simulink model "washout2useful"  (R2018b)
settings: Solver=VariableStepAuto  StartTime=0.0  StopTime=30  RelTol=1e-3
undefined symbols (not defined in the file or in its folder): sigbuilder_block
settings Model: Creator=15705  LastModifiedBy=15705

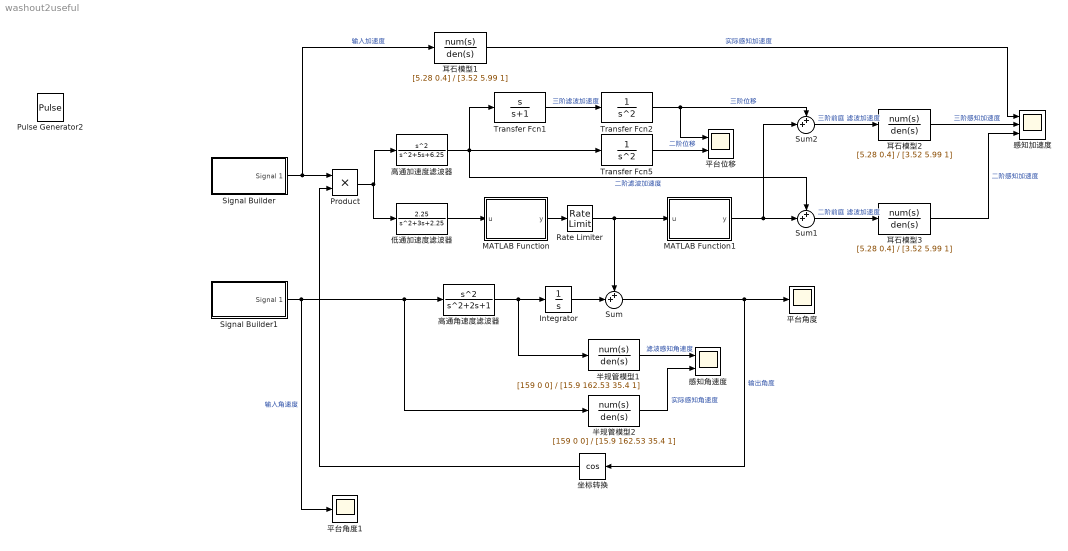
== system washout2useful ==
  Integrator : Integrator
  MATLAB Function : MATLAB Function  TreatAsAtomicUnit=on
  MATLAB Function1 : MATLAB Function  TreatAsAtomicUnit=on
  Product : Product
  Pulse Generator2 : DiscretePulseGenerator  PulseType=Time based  Period=10  PulseWidth=50  PhaseDelay=2
  Rate Limiter : RateLimiter  RisingSlewLimit=0.0628  FallingSlewLimit=-0.0628  SampleTimeMode=inherited
  Signal Builder : Subsystem  Tag=STV Subsys  LoadFcn=sigbuilder_block('load');  StartFcn=sigbuilder_block('start');  StopFcn=sigbuilder_block('stop');  ClipboardFcn=sigbuilder_block('clipboard');  mask(Sigbuilder block){tuvar=[0:10]}
      mask help: Simulink:masks:SigbuilderBlock_MD
      mask init:
      | if ~strcmp(get_param(bdroot(gcbh),'SimulationStatus'),'stopped') tuvar = sigbuilder_block('maskInit'); end
      settings: CopyFcn=sigbuilder_block('copy');  DeleteFcn=sigbuilder_block('delete');  ModelCloseFcn=sigbuilder_block('modelClose');  PreSaveFcn=sigbuilder_block('preSave');  PauseFcn=sigbuilder_block('pause');  ContinueFcn=sigbuilder_block('continue');  NameChangeFcn=sigbuilder_block('namechange');  OpenFcn=sigbuilder_block('open',[294.375 70.5 550.5 364.5 ]);  CloseFcn=sigbuilder_block('close');
      mask Display: plot(0, 0, 100, 100,[2, 2, 32, 32, 2], [68, 8, 8, 68, 68],[32, 2], [38, 38], [32, 19, 2],[53, 60, 44], [32, 17, 17, 2],[16, 16, 31, 31]);txt = getActiveGroup(gcbh);text(2, 100, txt,'verticalAlignment', 'top');
  Signal Builder1 : Subsystem  Tag=STV Subsys  LoadFcn=sigbuilder_block('load');  StartFcn=sigbuilder_block('start');  StopFcn=sigbuilder_block('stop');  ClipboardFcn=sigbuilder_block('clipboard');  mask(Sigbuilder block){tuvar=[0:10]}
      mask help: Simulink:masks:SigbuilderBlock_MD
      mask init:
      | if ~strcmp(get_param(bdroot(gcbh),'SimulationStatus'),'stopped') tuvar = sigbuilder_block('maskInit'); end
      settings: CopyFcn=sigbuilder_block('copy');  DeleteFcn=sigbuilder_block('delete');  ModelCloseFcn=sigbuilder_block('modelClose');  PreSaveFcn=sigbuilder_block('preSave');  PauseFcn=sigbuilder_block('pause');  ContinueFcn=sigbuilder_block('continue');  NameChangeFcn=sigbuilder_block('namechange');  OpenFcn=sigbuilder_block('open',[294.375 70.5 550.5 364.5 ]);  CloseFcn=sigbuilder_block('close');
      mask Display: plot(0, 0, 100, 100,[2, 2, 32, 32, 2], [68, 8, 8, 68, 68],[32, 2], [38, 38], [32, 19, 2],[53, 60, 44], [32, 17, 17, 2],[16, 16, 31, 31]);txt = getActiveGroup(gcbh);text(2, 100, txt,'verticalAlignment', 'top');
  Sum : Sum  Inputs=++|
  Sum1 : Sum  Inputs=++|
  Sum2 : Sum  Inputs=++|
  Transfer Fcn1 : TransferFcn  Numerator=[1 0]  Denominator=[1 1]
  Transfer Fcn2 : TransferFcn  Denominator=[1 0 0]
  Transfer Fcn5 : TransferFcn  Denominator=[1 0 0]
  低通加速度滤波器 : TransferFcn  Numerator=[2.25]  Denominator=[1 3 2.25]
  半规管模型1 : TransferFcn  Numerator=[159 0 0]  Denominator=[15.9 162.53 35.4 1]
  半规管模型2 : TransferFcn  Numerator=[159 0 0]  Denominator=[15.9 162.53 35.4 1]
  坐标转换 : Trigonometry  Operator=cos
  平台位移 : Scope  NumInputPorts=2
  平台角度 : Scope
  平台角度1 : Scope
  感知加速度 : Scope  NumInputPorts=3
  感知角速度 : Scope  NumInputPorts=2
  耳石模型1 : TransferFcn  Numerator=[5.28 0.4]  Denominator=[3.52 5.99 1]
  耳石模型2 : TransferFcn  Numerator=[5.28 0.4]  Denominator=[3.52 5.99 1]
  耳石模型3 : TransferFcn  Numerator=[5.28 0.4]  Denominator=[3.52 5.99 1]
  高通加速度滤波器 : TransferFcn  Numerator=[1 0 0]  Denominator=[1 5 6.25]
  高通角速度滤波器 : TransferFcn  Numerator=[1 0 0]
  wires:
  Signal Builder/1(Signal 1) -> Product/1, 耳石模型1/1  "输入加速度"
  高通加速度滤波器/1 -> Transfer Fcn1/1, Sum1/1, Transfer Fcn5/1  "二阶滤波加速度"
  Transfer Fcn1/1 -> Transfer Fcn2/1  "三阶滤波加速度"
  MATLAB Function/1(y) -> Rate Limiter/1
  高通角速度滤波器/1 -> 半规管模型1/1, Integrator/1
  Rate Limiter/1 -> MATLAB Function1/1(u), Sum/1
  Integrator/1 -> Sum/2
  Transfer Fcn5/1 -> 平台位移/2  "二阶位移"
  Transfer Fcn2/1 -> Sum2/1, 平台位移/1  "三阶位移"
  低通加速度滤波器/1 -> MATLAB Function/1(u)
  Signal Builder1/1(Signal 1) -> 平台角度1/1, 半规管模型2/1, 高通角速度滤波器/1  "输入角速度"
  Sum/1 -> 坐标转换/1, 平台角度/1  "输出角度"
  Sum1/1 -> 耳石模型3/1  "二阶前庭 滤波加速度"
  Sum2/1 -> 耳石模型2/1  "三阶前庭 滤波加速度"
  耳石模型1/1 -> 感知加速度/1  "实际感知加速度"
  耳石模型2/1 -> 感知加速度/2  "三阶感知加速度"
  耳石模型3/1 -> 感知加速度/3  "二阶感知加速度"
  MATLAB Function1/1(y) -> Sum2/2, Sum1/2
  半规管模型1/1 -> 感知角速度/1  "滤波感知角速度"
  半规管模型2/1 -> 感知角速度/2  "实际感知角速度"
  Product/1 -> 低通加速度滤波器/1, 高通加速度滤波器/1
  坐标转换/1 -> Product/2

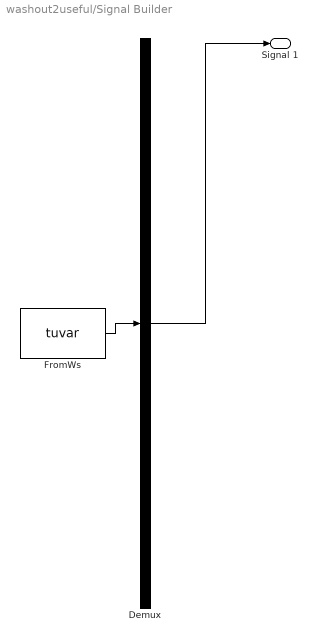
== system washout2useful/Signal Builder ==
  Demux : Demux  Tag=STV Demux  Outputs=1
  FromWs : FromWorkspace  Tag=STV FromWs  VariableName=tuvar  SampleTime=0
      SigBuilderData=|
      | common.afterFinalStr = 'Extrapolate'
      | common.sampleTime = 0
      | dataSet.timeRange = [0 10]
      | dataSet.name = 'Group 1'
      | sbobj.Groups.Name = 'Group 1'
      | sbobj.Groups.Signals.Name = 'Signal 1'
      | sbobj.Groups.Signals.XData = [0 2 4 8 8 10]
      | sbobj.Groups.Signals.YData = [-0.005 -0.005 1 1.005 0 0]
  Signal 1 : Outport  Tag=STV Outport
  wires:
  Demux/1 -> Signal 1/1
  FromWs/1 -> Demux/1

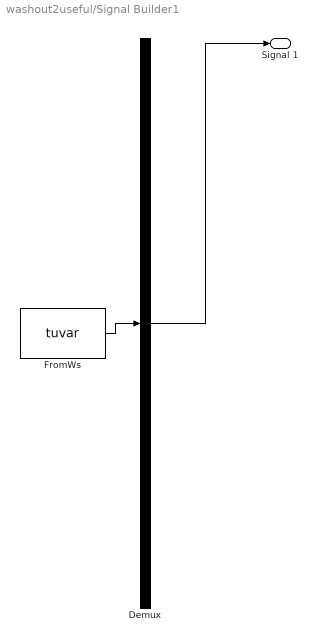
== system washout2useful/Signal Builder1 ==
  Demux : Demux  Tag=STV Demux  Outputs=1
  FromWs : FromWorkspace  Tag=STV FromWs  VariableName=tuvar  SampleTime=0
      SigBuilderData=|
      | common.afterFinalStr = 'Extrapolate'
      | common.sampleTime = 0
      | dataSet.timeRange = [0 10]
      | dataSet.name = 'Group 1'
      | sbobj.Groups.Name = 'Group 1'
      | sbobj.Groups.Signals.Name = 'Signal 1'
      | sbobj.Groups.Signals.XData = [0 2 4 8 8 10]
      | sbobj.Groups.Signals.YData = [-0.005 -0.005 1 1.005 0 0]
  Signal 1 : Outport  Tag=STV Outport
  wires:
  Demux/1 -> Signal 1/1
  FromWs/1 -> Demux/1

== matlab function washout2useful/MATLAB Function1 ==
  data: u input; y output
function y = fcn(u)
y=9.8*sin(u);

== matlab function washout2useful/MATLAB Function ==
  data: u input; y output
function y = fcn(u)
y=asin(u/9.8);
